simulink model "problema5"  (R2018a)
settings: Solver=VariableStepAuto  StartTime=0.0  StopTime=10.0  RelTol=1e-3
undefined symbols (not defined in the file): D, N, s
settings Model: Creator=Migue  LastModifiedBy=Migue

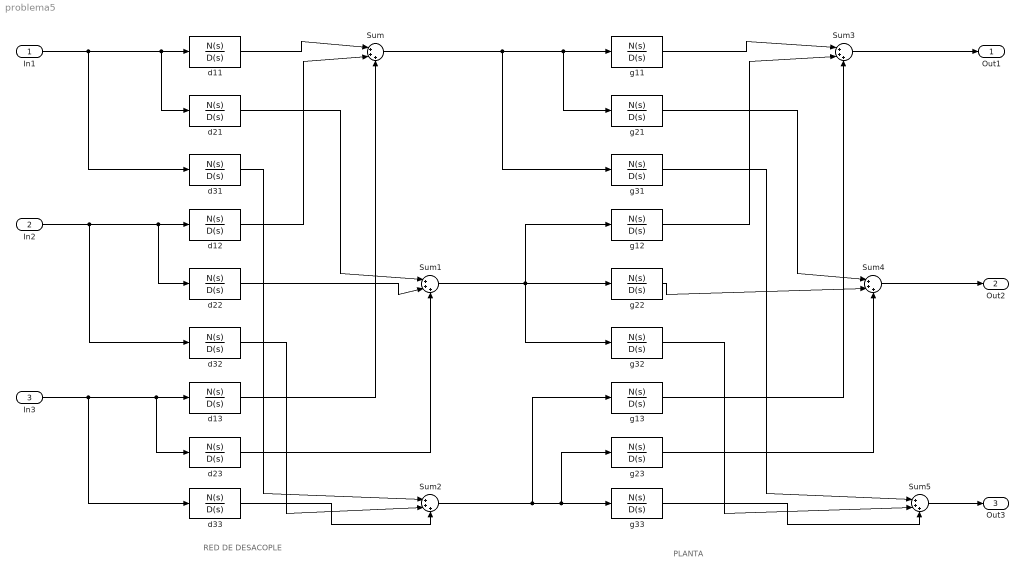
== system problema5 ==
  note: RED DE DESACOPLE
  note: PLANTA
  In1 : Inport
  In2 : Inport  Port=2
  In3 : Inport  Port=3
  Sum{,1..5} (6 alike) : Sum  Inputs=|+++
  d{11..13,21..23,31..33} (9 alike) : TransferFcn  Numerator=N(s)  Denominator=D(s)  ContinuousStateAttributes="''da\""
  g{11..13,21..23,31..33} (9 alike) : TransferFcn  Numerator=N(s)  Denominator=D(s)  ContinuousStateAttributes="''da\""
  Out1 : Outport
  Out2 : Outport  Port=2
  Out3 : Outport  Port=3
  wires:
  In1/1 -> d31/1, d21/1, d11/1
  In2/1 -> d32/1, d22/1, d12/1
  In3/1 -> d33/1, d23/1, d13/1
  d11/1 -> Sum/1
  d12/1 -> Sum/2
  d13/1 -> Sum/3
  d21/1 -> Sum1/1
  d22/1 -> Sum1/2
  d23/1 -> Sum1/3
  d33/1 -> Sum2/3
  d32/1 -> Sum2/2
  d31/1 -> Sum2/1
  Sum/1 -> g31/1, g21/1, g11/1
  Sum1/1 -> g32/1, g22/1, g12/1
  Sum2/1 -> g13/1, g23/1, g33/1
  g11/1 -> Sum3/1
  g12/1 -> Sum3/2
  g13/1 -> Sum3/3
  g21/1 -> Sum4/1
  g22/1 -> Sum4/2
  g23/1 -> Sum4/3
  g33/1 -> Sum5/3
  g32/1 -> Sum5/2
  g31/1 -> Sum5/1
  Sum3/1 -> Out1/1
  Sum4/1 -> Out2/1
  Sum5/1 -> Out3/1
